simulink model "ADU_Integration_Y2016_simulation"  (R2016b)
settings: Solver=FixedStepDiscrete  StartTime=240  StopTime=300  FixedStep=0.01  RelTol=1e-3  EnableMultiTasking=on
PostLoadFcn:
  | , if any(exist('dsrtsu_mdlpostloadfcn', 'file') == [2, 3, 6]), try dsrtsu_mdlpostloadfcn('Execute', bdroot); catch fprintf('Error in PostLoadFcn (dsrtsu_mdlpostloadfcn) for model "%s":\n %s\n', bdroot, lasterr); end, end,
InitFcn:
  | load 'data/chi2_dat';
  | load 'data/innerLine_struct';
  | load 'data/middleLine_struct';
  | load 'data/outerLine_struct';
  | load 'data/innerLine';
  | load 'data/middleLine';
  | load 'data/outerLine';
  | load 'data/landmarks_patac_schimmel_ccw';
  | load 'data/patac_navi_array';
  | load 'data/sensor';
  | load 'data/map_struct';
  | addpath map_src
  | Integration_Parameter;
  | load 'TestData_001';
values from neighbouring files (symbols this model uses):
  TestData_001 =     [TestData_001.mat]
undefined symbols (not defined in the file or in its folder): a, chi2_dat, innerLine, landmarks_patac_schimmel_ccw, middleLine, outerLine, patac_navi_array, StartNum
libraries: simulink x36, rtican x1
(part 8 of 20)

== system ADU_Integration_Y2016_simulation/Fusion_Model/Fusion_Block/Side_Fusion/Side_Fusion/Tracker_Update.Tracker_Filter.Update.Update ==
  Pre_x : Inport
  Pre_vx : Inport  Port=2
  Pre_y : Inport  Port=3
  Pre_vy : Inport  Port=4
  pre_p11 : Inport  Port=5
  pre_p12 : Inport  Port=6
  pre_p13 : Inport  Port=7
  pre_p14 : Inport  Port=8
  pre_p21 : Inport  Port=9
  pre_p22 : Inport  Port=10
  pre_p23 : Inport  Port=11
  pre_p24 : Inport  Port=12
  pre_p31 : Inport  Port=13
  pre_p32 : Inport  Port=14
  pre_p33 : Inport  Port=15
  pre_p34 : Inport  Port=16
  pre_p41 : Inport  Port=17
  pre_p42 : Inport  Port=18
  pre_p43 : Inport  Port=19
  pre_p44 : Inport  Port=20
  mk : Inport  Port=21
  m00 : Inport  Port=22
  m01 : Inport  Port=23
  m2 : Inport  Port=24
  m10 : Inport  Port=25
  m11 : Inport  Port=26
  m12 : Inport  Port=27
  m20 : Inport  Port=28
  m21 : Inport  Port=29
  m22 : Inport  Port=30
  Pt0 : Inport  Port=31
  f : TriggerPort  TriggerType=function-call  VariantControl=Variant
      settings: CopyFcn=Stateflow.SLINSF.SimulinkMan.removeBlockPreDeleteFcn  PreDeleteFcn=Stateflow.SLINSF.SimulinkMan.unsafePredeleteFcn
  Model_Update : Subsystem
  RangeX : Outport
  VelX : Outport  Port=2
  RangeY : Outport  Port=3
  VelY : Outport  Port=4
  P11 : Outport  Port=5
  P12 : Outport  Port=6
  P13 : Outport  Port=7
  P14 : Outport  Port=8
  P21 : Outport  Port=9
  P22 : Outport  Port=10
  P23 : Outport  Port=11
  P24 : Outport  Port=12
  P31 : Outport  Port=13
  P32 : Outport  Port=14
  P33 : Outport  Port=15
  P34 : Outport  Port=16
  P41 : Outport  Port=17
  P42 : Outport  Port=18
  P43 : Outport  Port=19
  P44 : Outport  Port=20
  wires:
  Model_Update/1(RangeX) -> RangeX/1
  Model_Update/2(VelX) -> VelX/1
  Model_Update/3(RangeY) -> RangeY/1
  Model_Update/4(VelY) -> VelY/1
  Model_Update/5(P11) -> P11/1
  Model_Update/6(P12) -> P12/1
  Model_Update/7(P13) -> P13/1
  Model_Update/8(P14) -> P14/1
  Model_Update/9(P21) -> P21/1
  Model_Update/10(P22) -> P22/1
  Model_Update/11(P23) -> P23/1
  Model_Update/12(P24) -> P24/1
  Model_Update/13(P31) -> P31/1
  Model_Update/14(P32) -> P32/1
  Model_Update/15(P33) -> P33/1
  Model_Update/16(P34) -> P34/1
  Model_Update/17(P41) -> P41/1
  Model_Update/18(P42) -> P42/1
  Model_Update/19(P43) -> P43/1
  Model_Update/20(P44) -> P44/1
  pre_p41/1 -> Model_Update/17(pre_p41)
  pre_p33/1 -> Model_Update/15(pre_p33)
  pre_p34/1 -> Model_Update/16(pre_p34)
  pre_p42/1 -> Model_Update/18(pre_p42)
  pre_p24/1 -> Model_Update/12(pre_p24)
  pre_p31/1 -> Model_Update/13(pre_p31)
  pre_p32/1 -> Model_Update/14(pre_p32)
  mk/1 -> Model_Update/21(mk)  "Measurement_Num"
  pre_p22/1 -> Model_Update/10(pre_p22)
  pre_p43/1 -> Model_Update/19(pre_p43)
  pre_p44/1 -> Model_Update/20(pre_p44)
  pre_p23/1 -> Model_Update/11(pre_p23)
  pre_p21/1 -> Model_Update/9(pre_p21)
  pre_p11/1 -> Model_Update/5(pre_p11)
  Pre_y/1 -> Model_Update/3(Pre_y)  "Pre_y"
  Pre_x/1 -> Model_Update/1(Pre_x)  "Pre_x"
  Pre_vx/1 -> Model_Update/2(Pre_vx)  "Pre_vx"
  Pre_vy/1 -> Model_Update/4(Pre_vy)  "Pre_vy"
  pre_p12/1 -> Model_Update/6(pre_p12)
  pre_p13/1 -> Model_Update/7(pre_p13)
  pre_p14/1 -> Model_Update/8(pre_p14)
  m00/1 -> Model_Update/22(m00)  "Measurement_1_Possible"
  m12/1 -> Model_Update/27(m12)  "Measurement_2_Y_Error"
  m2/1 -> Model_Update/24(m2)  "Measurement_1_Y_Error"
  m11/1 -> Model_Update/26(m11)  "Measurement_2_X_Error"
  m10/1 -> Model_Update/25(m10)  "Measurement_2_Possible"
  m01/1 -> Model_Update/23(m01)  "Measurement_1_X_Error"
  m20/1 -> Model_Update/28(m20)  "Measurement_3_Possible"
  m22/1 -> Model_Update/30(m22)  "Measurement_3_Y_Error"
  m21/1 -> Model_Update/29(m21)  "Measurement_3_X_Error"
  Pt0/1 -> Model_Update/31(Pt0)

== system ADU_Integration_Y2016_simulation/Fusion_Model/Fusion_Block/Global_Fusion/Fusion_Center/FusTrackPredict.Forecast/No_Zero1 ==
  In : Inport
  Abs : Abs
  Compare To Constant : simulink/Logic and Bit Operations/Compare To Constant  relop=>=  const=0.001  OutDataTypeStr=uint8
  Constant : Constant  Value=0.001
  Switch : Switch  Threshold=0.5
  Out : Outport
  wires:
  Constant/1 -> Switch/3
  Switch/1 -> Out/1
  Compare To Constant/1 -> Switch/2
  In/1 -> Switch/1, Abs/1
  Abs/1 -> Compare To Constant/1

== system ADU_Integration_Y2016_simulation/Fusion_Model/Fusion_Block/Global_Fusion/Fusion_Center/FusTrackPredict.Forecast/No_Zero2 ==
  In : Inport
  Abs : Abs
  Compare To Constant : simulink/Logic and Bit Operations/Compare To Constant  relop=>=  const=0.001  OutDataTypeStr=uint8
  Constant : Constant  Value=0.001
  Switch : Switch  Threshold=0.5
  Out : Outport
  wires:
  Abs/1 -> Compare To Constant/1
  In/1 -> Abs/1, Switch/1
  Compare To Constant/1 -> Switch/2
  Switch/1 -> Out/1
  Constant/1 -> Switch/3

== system ADU_Integration_Y2016_simulation/Fusion_Model/Fusion_Block/Global_Fusion/Fusion_Center/FusTrackPredict.Forecast/No_Zero3 ==
  In : Inport
  Abs : Abs
  Compare To Constant : simulink/Logic and Bit Operations/Compare To Constant  relop=>=  const=0.001  OutDataTypeStr=uint8
  Constant : Constant  Value=0.001
  Switch : Switch  Threshold=0.5
  Out : Outport
  wires:
  Constant/1 -> Switch/3
  Switch/1 -> Out/1
  Compare To Constant/1 -> Switch/2
  In/1 -> Switch/1, Abs/1
  Abs/1 -> Compare To Constant/1

== system ADU_Integration_Y2016_simulation/Fusion_Model/Fusion_Block/Global_Fusion/Fusion_Center/FusTrackPredict.Forecast/No_Zero4 ==
  In : Inport
  Abs : Abs
  Compare To Constant : simulink/Logic and Bit Operations/Compare To Constant  relop=>=  const=0.001  OutDataTypeStr=uint8
  Constant : Constant  Value=0.001
  Switch : Switch  Threshold=0.5
  Out : Outport
  wires:
  Abs/1 -> Compare To Constant/1
  In/1 -> Abs/1, Switch/1
  Compare To Constant/1 -> Switch/2
  Switch/1 -> Out/1
  Constant/1 -> Switch/3

== system ADU_Integration_Y2016_simulation/Fusion_Model/Fusion_Block/Global_Fusion/Fusion_Center/FusTrackPredict.Forecast/P_Gen ==
  pre_p11 : Inport
  pre_p12 : Inport  Port=2
  pre_p13 : Inport  Port=3
  pre_p14 : Inport  Port=4
  pre_p21 : Inport  Port=5
  pre_p22 : Inport  Port=6
  pre_p23 : Inport  Port=7
  pre_p24 : Inport  Port=8
  pre_p31 : Inport  Port=9
  pre_p32 : Inport  Port=10
  pre_p33 : Inport  Port=11
  pre_p34 : Inport  Port=12
  pre_p41 : Inport  Port=13
  pre_p42 : Inport  Port=14
  pre_p43 : Inport  Port=15
  pre_p44 : Inport  Port=16
  Add : Sum  Inputs=++++
  Gain : Gain  Gain=[1;0;0;0]  Multiplication=Matrix(K*u)
  Gain1 : Gain  Gain=[0;1;0;0]  Multiplication=Matrix(K*u)
  Gain2 : Gain  Gain=[0;0;1;0]  Multiplication=Matrix(K*u)
  Gain3 : Gain  Gain=[0;0;0;1]  Multiplication=Matrix(K*u)
  Math Function{1..4} (4 alike) : Math  Operator=transpose  SaturateOnIntegerOverflow=on
  Mux{,1..3} (4 alike) : Mux
  P_Pre[4x4] : Outport
  wires:
  Mux/1 -> Math Function2/1
  Math Function2/1 -> Gain/1
  Mux1/1 -> Math Function1/1
  Math Function1/1 -> Gain1/1
  Mux2/1 -> Math Function4/1
  Math Function4/1 -> Gain2/1
  Mux3/1 -> Math Function3/1
  Math Function3/1 -> Gain3/1
  Gain/1 -> Add/1
  Gain1/1 -> Add/2
  Gain2/1 -> Add/3
  Gain3/1 -> Add/4
  pre_p11/1 -> Mux/1
  pre_p12/1 -> Mux/2
  pre_p13/1 -> Mux/3
  pre_p14/1 -> Mux/4
  pre_p21/1 -> Mux1/1
  pre_p22/1 -> Mux1/2
  pre_p23/1 -> Mux1/3
  pre_p24/1 -> Mux1/4
  pre_p31/1 -> Mux2/1
  pre_p32/1 -> Mux2/2
  pre_p33/1 -> Mux2/3
  pre_p34/1 -> Mux2/4
  pre_p41/1 -> Mux3/1
  pre_p42/1 -> Mux3/2
  pre_p43/1 -> Mux3/3
  pre_p44/1 -> Mux3/4
  Add/1 -> P_Pre[4x4]/1

== system ADU_Integration_Y2016_simulation/Fusion_Model/Fusion_Block/Global_Fusion/Fusion_Center/FusTrackPredict.Forecast/Predict ==
  DataIn : Inport
  Bus Creator1 : BusCreator  Inputs=2
  F : Subsystem
  State_PreTime : Subsystem
  DataOut : Outport
  wires:
  DataIn/1 -> F/1(DataIn), State_PreTime/1(Source)  "Z_Mea"
  State_PreTime/1(X_k) -> Bus Creator1/1  "X_k[4x1]"
  F/1(F) -> Bus Creator1/2  "F[4x4]"
  Bus Creator1/1 -> DataOut/1

== system ADU_Integration_Y2016_simulation/Fusion_Model/Fusion_Block/Global_Fusion/Fusion_Center/FusTrackPredict.Forecast/Predict_X_P ==
  In : Inport
  P_k : Inport  Port=2
  Bus Creator : BusCreator  Inputs=3
  Bus Selector : BusSelector  OutputSignals=F[4x4],X_k[4x1]
  Bus Selector1 : BusSelector  OutputSignals=F[4x4],F[4x4]
  Math Function : Math  Operator=transpose  SaturateOnIntegerOverflow=on
  Product : Product  Multiplication=Matrix(*)  RndMeth=Zero
  Product1 : Product  Inputs=3  Multiplication=Matrix(*)  RndMeth=Zero
  Q : Constant  Value=[0.01 0 0 0;0 0.01 0 0;0 0 0.01 0;0 0 0 0.01]
  Subtract2 : Sum
  DataOut : Outport
  wires:
  In/1 -> Bus Selector/1, Bus Selector1/1, Bus Creator/3  "Signal_temp"
  Bus Selector/1 -> Product/1  "<F[4x4]>"
  Bus Selector/2 -> Product/2  "<X_k[4x1]>"
  P_k/1 -> Product1/2
  Bus Selector1/1 -> Product1/1  "<F[4x4]>"
  Bus Selector1/2 -> Math Function/1  "<F[4x4]>"
  Math Function/1 -> Product1/3
  Product/1 -> Bus Creator/1  "x_predict[4x1]"
  Subtract2/1 -> Bus Creator/2  "P_predict"
  Bus Creator/1 -> DataOut/1
  Product1/1 -> Subtract2/1  "P_predict"
  Q/1 -> Subtract2/2

== system ADU_Integration_Y2016_simulation/Fusion_Model/Fusion_Block/Global_Fusion/Fusion_Center/FusTrackUpdate.MDCal/No_Zero1 ==
  In : Inport
  Abs : Abs
  Compare To Constant : simulink/Logic and Bit Operations/Compare To Constant  relop=>=  const=0.001  OutDataTypeStr=uint8
  Constant : Constant  Value=0.001
  Switch : Switch  Threshold=0.5
  Out : Outport
  wires:
  Constant/1 -> Switch/3
  Switch/1 -> Out/1
  Compare To Constant/1 -> Switch/2
  In/1 -> Switch/1, Abs/1
  Abs/1 -> Compare To Constant/1

== system ADU_Integration_Y2016_simulation/Fusion_Model/Fusion_Block/Global_Fusion/Fusion_Center/FusTrackUpdate.MDCal/No_Zero2 ==
  In : Inport
  Abs : Abs
  Compare To Constant : simulink/Logic and Bit Operations/Compare To Constant  relop=>=  const=0.001  OutDataTypeStr=uint8
  Constant : Constant  Value=0.001
  Switch : Switch  Threshold=0.5
  Out : Outport
  wires:
  Abs/1 -> Compare To Constant/1
  In/1 -> Abs/1, Switch/1
  Compare To Constant/1 -> Switch/2
  Switch/1 -> Out/1
  Constant/1 -> Switch/3

== system ADU_Integration_Y2016_simulation/Fusion_Model/Fusion_Block/Global_Fusion/Fusion_Center/FusTrackUpdate.MDCal/No_Zero3 ==
  In : Inport
  Abs : Abs
  Compare To Constant : simulink/Logic and Bit Operations/Compare To Constant  relop=>=  const=0.001  OutDataTypeStr=uint8
  Constant : Constant  Value=0.001
  Switch : Switch  Threshold=0.5
  Out : Outport
  wires:
  Constant/1 -> Switch/3
  Switch/1 -> Out/1
  Compare To Constant/1 -> Switch/2
  In/1 -> Switch/1, Abs/1
  Abs/1 -> Compare To Constant/1

== system ADU_Integration_Y2016_simulation/Fusion_Model/Fusion_Block/Global_Fusion/Fusion_Center/FusTrackUpdate.MDCal/No_Zero4 ==
  In : Inport
  Abs : Abs
  Compare To Constant : simulink/Logic and Bit Operations/Compare To Constant  relop=>=  const=0.001  OutDataTypeStr=uint8
  Constant : Constant  Value=0.001
  Switch : Switch  Threshold=0.5
  Out : Outport
  wires:
  Abs/1 -> Compare To Constant/1
  In/1 -> Abs/1, Switch/1
  Compare To Constant/1 -> Switch/2
  Switch/1 -> Out/1
  Constant/1 -> Switch/3

== system ADU_Integration_Y2016_simulation/Fusion_Model/Fusion_Block/Global_Fusion/Fusion_Center/FusTrackUpdate.MDCal/Subsystem ==
  R11 : Inport
  R12 : Inport  Port=2
  R21 : Inport  Port=3
  R22 : Inport  Port=4
  Add : Sum
  Gain : Gain  Gain=[1;0]  Multiplication=Matrix(K*u)
  Gain1 : Gain  Gain=[0;1]  Multiplication=Matrix(K*u)
  Math Function1 : Math  Operator=transpose  SaturateOnIntegerOverflow=on
  Math Function2 : Math  Operator=transpose  SaturateOnIntegerOverflow=on
  Mux2 : Mux  Inputs=2
  Mux3 : Mux  Inputs=2
  R[2x2] : Outport
  wires:
  R21/1 -> Mux3/1
  Gain1/1 -> Add/2
  Math Function1/1 -> Gain1/1
  R22/1 -> Mux3/2
  Mux3/1 -> Math Function1/1
  Mux2/1 -> Math Function2/1
  Gain/1 -> Add/1
  Math Function2/1 -> Gain/1
  Add/1 -> R[2x2]/1
  R11/1 -> Mux2/1
  R12/1 -> Mux2/2

== system ADU_Integration_Y2016_simulation/Fusion_Model/Fusion_Block/Global_Fusion/Fusion_Center/FusTrackUpdate.MDCal/W_Gen ==
  R11 : Inport
  R12 : Inport  Port=2
  R13 : Inport  Port=3
  R14 : Inport  Port=4
  R21 : Inport  Port=5
  R22 : Inport  Port=6
  R23 : Inport  Port=7
  R24 : Inport  Port=8
  R31 : Inport  Port=9
  R32 : Inport  Port=10
  R33 : Inport  Port=11
  R34 : Inport  Port=12
  R41 : Inport  Port=13
  R42 : Inport  Port=14
  R43 : Inport  Port=15
  R44 : Inport  Port=16
  Add : Sum  Inputs=++++
  Gain : Gain  Gain=[1;0;0;0]  Multiplication=Matrix(K*u)
  Gain1 : Gain  Gain=[0;1;0;0]  Multiplication=Matrix(K*u)
  Gain2 : Gain  Gain=[0;0;1;0]  Multiplication=Matrix(K*u)
  Gain3 : Gain  Gain=[0;0;0;1]  Multiplication=Matrix(K*u)
  Math Function{1..4} (4 alike) : Math  Operator=transpose  SaturateOnIntegerOverflow=on
  Mux{,1..3} (4 alike) : Mux
  P_Pre : Outport
  wires:
  Mux/1 -> Math Function2/1
  Math Function2/1 -> Gain/1
  Mux1/1 -> Math Function1/1
  Math Function1/1 -> Gain1/1
  Mux2/1 -> Math Function4/1
  Math Function4/1 -> Gain2/1
  Mux3/1 -> Math Function3/1
  Math Function3/1 -> Gain3/1
  Gain/1 -> Add/1
  Gain1/1 -> Add/2
  Gain2/1 -> Add/3
  Gain3/1 -> Add/4
  R11/1 -> Mux/1
  R12/1 -> Mux/2
  R13/1 -> Mux/3
  R14/1 -> Mux/4
  R21/1 -> Mux1/1
  R22/1 -> Mux1/2
  R23/1 -> Mux1/3
  R24/1 -> Mux1/4
  R31/1 -> Mux2/1
  R32/1 -> Mux2/2
  R33/1 -> Mux2/3
  R34/1 -> Mux2/4
  R41/1 -> Mux3/1
  R42/1 -> Mux3/2
  R43/1 -> Mux3/3
  R44/1 -> Mux3/4
  Add/1 -> P_Pre/1

== system ADU_Integration_Y2016_simulation/Fusion_Model/Fusion_Block/Global_Fusion/Fusion_Center/FusTrackUpdate.Update/No_Zero1 ==
  In : Inport
  Abs : Abs
  Compare To Constant : simulink/Logic and Bit Operations/Compare To Constant  relop=>=  const=0.001  OutDataTypeStr=uint8
  Constant : Constant  Value=0.001
  Switch : Switch  Threshold=0.5
  Out : Outport
  wires:
  Abs/1 -> Compare To Constant/1
  In/1 -> Abs/1, Switch/1
  Compare To Constant/1 -> Switch/2
  Switch/1 -> Out/1
  Constant/1 -> Switch/3

== system ADU_Integration_Y2016_simulation/Fusion_Model/Fusion_Block/Global_Fusion/Fusion_Center/FusTrackUpdate.Update/No_Zero2 ==
  In : Inport
  Abs : Abs
  Compare To Constant : simulink/Logic and Bit Operations/Compare To Constant  relop=>=  const=0.001  OutDataTypeStr=uint8
  Constant : Constant  Value=0.001
  Switch : Switch  Threshold=0.5
  Out : Outport
  wires:
  Constant/1 -> Switch/3
  Switch/1 -> Out/1
  Compare To Constant/1 -> Switch/2
  In/1 -> Switch/1, Abs/1
  Abs/1 -> Compare To Constant/1

== system ADU_Integration_Y2016_simulation/Fusion_Model/Fusion_Block/Global_Fusion/Fusion_Center/FusTrackUpdate.Update/No_Zero3 ==
  In : Inport
  Abs : Abs
  Compare To Constant : simulink/Logic and Bit Operations/Compare To Constant  relop=>=  const=0.001  OutDataTypeStr=uint8
  Constant : Constant  Value=0.001
  Switch : Switch  Threshold=0.5
  Out : Outport
  wires:
  Abs/1 -> Compare To Constant/1
  In/1 -> Abs/1, Switch/1
  Compare To Constant/1 -> Switch/2
  Switch/1 -> Out/1
  Constant/1 -> Switch/3

== system ADU_Integration_Y2016_simulation/Fusion_Model/Fusion_Block/Global_Fusion/Fusion_Center/FusTrackUpdate.Update/No_Zero4 ==
  In : Inport
  Abs : Abs
  Compare To Constant : simulink/Logic and Bit Operations/Compare To Constant  relop=>=  const=0.001  OutDataTypeStr=uint8
  Constant : Constant  Value=0.001
  Switch : Switch  Threshold=0.5
  Out : Outport
  wires:
  Constant/1 -> Switch/3
  Switch/1 -> Out/1
  Compare To Constant/1 -> Switch/2
  In/1 -> Switch/1, Abs/1
  Abs/1 -> Compare To Constant/1

== system ADU_Integration_Y2016_simulation/Fusion_Model/Fusion_Block/Global_Fusion/Fusion_Center/FusTrackUpdate.Update/P_Gen ==
  pre_p11 : Inport
  pre_p12 : Inport  Port=2
  pre_p13 : Inport  Port=3
  pre_p14 : Inport  Port=4
  pre_p21 : Inport  Port=5
  pre_p22 : Inport  Port=6
  pre_p23 : Inport  Port=7
  pre_p24 : Inport  Port=8
  pre_p31 : Inport  Port=9
  pre_p32 : Inport  Port=10
  pre_p33 : Inport  Port=11
  pre_p34 : Inport  Port=12
  pre_p41 : Inport  Port=13
  pre_p42 : Inport  Port=14
  pre_p43 : Inport  Port=15
  pre_p44 : Inport  Port=16
  Add : Sum  Inputs=++++
  Gain : Gain  Gain=[1;0;0;0]  Multiplication=Matrix(K*u)
  Gain1 : Gain  Gain=[0;1;0;0]  Multiplication=Matrix(K*u)
  Gain2 : Gain  Gain=[0;0;1;0]  Multiplication=Matrix(K*u)
  Gain3 : Gain  Gain=[0;0;0;1]  Multiplication=Matrix(K*u)
  Math Function{1..4} (4 alike) : Math  Operator=transpose  SaturateOnIntegerOverflow=on
  Mux{,1..3} (4 alike) : Mux
  P_Pre : Outport
  wires:
  Mux/1 -> Math Function2/1
  Math Function2/1 -> Gain/1
  Mux1/1 -> Math Function1/1
  Math Function1/1 -> Gain1/1
  Mux2/1 -> Math Function4/1
  Math Function4/1 -> Gain2/1
  Mux3/1 -> Math Function3/1
  Math Function3/1 -> Gain3/1
  Gain/1 -> Add/1
  Gain1/1 -> Add/2
  Gain2/1 -> Add/3
  Gain3/1 -> Add/4
  pre_p11/1 -> Mux/1
  pre_p12/1 -> Mux/2
  pre_p13/1 -> Mux/3
  pre_p14/1 -> Mux/4
  pre_p21/1 -> Mux1/1
  pre_p22/1 -> Mux1/2
  pre_p23/1 -> Mux1/3
  pre_p24/1 -> Mux1/4
  pre_p31/1 -> Mux2/1
  pre_p32/1 -> Mux2/2
  pre_p33/1 -> Mux2/3
  pre_p34/1 -> Mux2/4
  pre_p41/1 -> Mux3/1
  pre_p42/1 -> Mux3/2
  pre_p43/1 -> Mux3/3
  pre_p44/1 -> Mux3/4
  Add/1 -> P_Pre/1

== system ADU_Integration_Y2016_simulation/Fusion_Model/Fusion_Block/Global_Fusion/Fusion_Center/FusTrackUpdate.Update/Predict ==
  DataIn : Inport
  Bus Creator1 : BusCreator  Inputs=3
  H : Constant  Value=[1 0 0 0;0 0 1 0]
  Measurement : Subsystem
  State_PreTime : Subsystem
  DataOut : Outport
  wires:
  DataIn/1 -> Measurement/1(Source), State_PreTime/1(Source)
  State_PreTime/1(X_k) -> Bus Creator1/1  "X_k"
  Measurement/1(Z_k) -> Bus Creator1/2  "Z_Mea"
  H/1 -> Bus Creator1/3  "H"
  Bus Creator1/1 -> DataOut/1

== system ADU_Integration_Y2016_simulation/Fusion_Model/Fusion_Block/Global_Fusion/Fusion_Center/FusTrackUpdate.Update/Predict_X_P ==
  In : Inport
  P_k : Inport  Port=2
  Bus Creator : BusCreator  Inputs=3
  Bus Selector : BusSelector  OutputSignals=X_k
  Gain : Gain
  DataOut : Outport
  wires:
  In/1 -> Bus Selector/1, Bus Creator/3  "Signal_temp"
  Bus Creator/1 -> DataOut/1
  Bus Selector/1 -> Gain/1  "<X_k>"
  P_k/1 -> Bus Creator/2  "P_predict"
  Gain/1 -> Bus Creator/1  "x_predict"

== system ADU_Integration_Y2016_simulation/Fusion_Model/Fusion_Block/Global_Fusion/Fusion_Center/FusTrackUpdate.Update/R_Cov_Gen ==
  R11 : Inport
  R12 : Inport  Port=2
  R21 : Inport  Port=3
  R22 : Inport  Port=4
  Add : Sum
  Gain : Gain  Gain=[1;0]  Multiplication=Matrix(K*u)
  Gain1 : Gain  Gain=[0;1]  Multiplication=Matrix(K*u)
  Math Function1 : Math  Operator=transpose  SaturateOnIntegerOverflow=on
  Math Function2 : Math  Operator=transpose  SaturateOnIntegerOverflow=on
  Mux : Mux  Inputs=2
  Mux1 : Mux  Inputs=2
  Cov_R_Measuerment : Outport
  wires:
  Add/1 -> Cov_R_Measuerment/1
  R22/1 -> Mux1/2
  R21/1 -> Mux1/1
  R12/1 -> Mux/2
  R11/1 -> Mux/1
  Gain1/1 -> Add/2
  Gain/1 -> Add/1
  Math Function1/1 -> Gain1/1
  Mux1/1 -> Math Function1/1
  Math Function2/1 -> Gain/1
  Mux/1 -> Math Function2/1

== system ADU_Integration_Y2016_simulation/Fusion_Model/Fusion_Block/Global_Fusion/Fusion_Center/FusTrackUpdate.Update/X_new ==
  note: 2X1
  note: 4X1
  note: 2X4
  note: 4X4
  note: 2X4
  note: 4X4
  note: 2X4
  W_k : Inport
  Data_In : Inport  Port=2
  Bus Selector : BusSelector  OutputSignals=P_predict,Signal_temp.H,Signal_temp.H,P_predict,Signal_temp.H
  Bus Selector1 : BusSelector  OutputSignals=Signal_temp.Z_Mea,Signal_temp.H,x_predict,x_predict
  Divide : Product  Inputs=*/  Multiplication=Matrix(*)
  Divide1 : Product  Inputs=**  Multiplication=Matrix(*)
  Divide2 : Product  Inputs=***  Multiplication=Matrix(*)
  Divide3 : Product  Inputs=**  Multiplication=Matrix(*)
  Divide4 : Product  Inputs=**  Multiplication=Matrix(*)
  Math Function : Math  Operator=transpose  SaturateOnIntegerOverflow=on
  Math Function1 : Math  Operator=transpose  SaturateOnIntegerOverflow=on
  Subtract : Sum
  Subtract1 : Sum
  Subtract2 : Sum  Inputs=+-
  X_update : Outport
  K : Outport  Port=2
  wires:
  Data_In/1 -> Bus Selector1/1, Bus Selector/1
  Bus Selector/1 -> Divide1/1  "<P_predict>"
  Bus Selector/2 -> Math Function1/1  "<H>"
  Bus Selector/5 -> Math Function/1  "<H>"
  Math Function/1 -> Divide2/3  "4X2"
  Bus Selector/4 -> Divide2/2  "<P_predict>"
  Bus Selector/3 -> Divide2/1  "<H>"
  Divide1/1 -> Divide/1  "4X2"
  Divide2/1 -> Subtract/1
  W_k/1 -> Subtract/2  "2X2"
  Subtract/1 -> Divide/2  "2X2"
  Bus Selector1/1 -> Subtract2/1  "<Z_Mea>"
  Bus Selector1/2 -> Divide3/1  "<H>"
  Divide3/1 -> Subtract2/2
  Bus Selector1/3 -> Divide3/2  "<x_predict>"
  Subtract2/1 -> Divide4/2
  Divide/1 -> Divide4/1, K/1  "K[4X2]"
  Divide4/1 -> Subtract1/1  "4X1"
  Bus Selector1/4 -> Subtract1/2  "<x_predict>"
  Subtract1/1 -> X_update/1
  Math Function1/1 -> Divide1/2  "4X2"

== system ADU_Integration_Y2016_simulation/Fusion_Model/Fusion_Block/Side_Fusion/Side_Fusion/FusTrackPredict.Forecast/No_Zero1 ==
  In : Inport
  Abs : Abs
  Compare To Constant : simulink/Logic and Bit Operations/Compare To Constant  relop=>=  const=0.001  OutDataTypeStr=uint8
  Constant : Constant  Value=0.001
  Switch : Switch  Threshold=0.5
  Out : Outport
  wires:
  Constant/1 -> Switch/3
  Switch/1 -> Out/1
  Compare To Constant/1 -> Switch/2
  In/1 -> Switch/1, Abs/1
  Abs/1 -> Compare To Constant/1

== system ADU_Integration_Y2016_simulation/Fusion_Model/Fusion_Block/Side_Fusion/Side_Fusion/FusTrackPredict.Forecast/No_Zero2 ==
  In : Inport
  Abs : Abs
  Compare To Constant : simulink/Logic and Bit Operations/Compare To Constant  relop=>=  const=0.001  OutDataTypeStr=uint8
  Constant : Constant  Value=0.001
  Switch : Switch  Threshold=0.5
  Out : Outport
  wires:
  Abs/1 -> Compare To Constant/1
  In/1 -> Abs/1, Switch/1
  Compare To Constant/1 -> Switch/2
  Switch/1 -> Out/1
  Constant/1 -> Switch/3

== system ADU_Integration_Y2016_simulation/Fusion_Model/Fusion_Block/Side_Fusion/Side_Fusion/FusTrackPredict.Forecast/No_Zero3 ==
  In : Inport
  Abs : Abs
  Compare To Constant : simulink/Logic and Bit Operations/Compare To Constant  relop=>=  const=0.001  OutDataTypeStr=uint8
  Constant : Constant  Value=0.001
  Switch : Switch  Threshold=0.5
  Out : Outport
  wires:
  Constant/1 -> Switch/3
  Switch/1 -> Out/1
  Compare To Constant/1 -> Switch/2
  In/1 -> Switch/1, Abs/1
  Abs/1 -> Compare To Constant/1

== system ADU_Integration_Y2016_simulation/Fusion_Model/Fusion_Block/Side_Fusion/Side_Fusion/FusTrackPredict.Forecast/No_Zero4 ==
  In : Inport
  Abs : Abs
  Compare To Constant : simulink/Logic and Bit Operations/Compare To Constant  relop=>=  const=0.001  OutDataTypeStr=uint8
  Constant : Constant  Value=0.001
  Switch : Switch  Threshold=0.5
  Out : Outport
  wires:
  Abs/1 -> Compare To Constant/1
  In/1 -> Abs/1, Switch/1
  Compare To Constant/1 -> Switch/2
  Switch/1 -> Out/1
  Constant/1 -> Switch/3

== system ADU_Integration_Y2016_simulation/Fusion_Model/Fusion_Block/Side_Fusion/Side_Fusion/FusTrackPredict.Forecast/P_Gen ==
  pre_p11 : Inport
  pre_p12 : Inport  Port=2
  pre_p13 : Inport  Port=3
  pre_p14 : Inport  Port=4
  pre_p21 : Inport  Port=5
  pre_p22 : Inport  Port=6
  pre_p23 : Inport  Port=7
  pre_p24 : Inport  Port=8
  pre_p31 : Inport  Port=9
  pre_p32 : Inport  Port=10
  pre_p33 : Inport  Port=11
  pre_p34 : Inport  Port=12
  pre_p41 : Inport  Port=13
  pre_p42 : Inport  Port=14
  pre_p43 : Inport  Port=15
  pre_p44 : Inport  Port=16
  Add : Sum  Inputs=++++
  Gain : Gain  Gain=[1;0;0;0]  Multiplication=Matrix(K*u)
  Gain1 : Gain  Gain=[0;1;0;0]  Multiplication=Matrix(K*u)
  Gain2 : Gain  Gain=[0;0;1;0]  Multiplication=Matrix(K*u)
  Gain3 : Gain  Gain=[0;0;0;1]  Multiplication=Matrix(K*u)
  Math Function{1..4} (4 alike) : Math  Operator=transpose  SaturateOnIntegerOverflow=on
  Mux{,1..3} (4 alike) : Mux
  P_Pre[4x4] : Outport
  wires:
  Mux/1 -> Math Function2/1
  Math Function2/1 -> Gain/1
  Mux1/1 -> Math Function1/1
  Math Function1/1 -> Gain1/1
  Mux2/1 -> Math Function4/1
  Math Function4/1 -> Gain2/1
  Mux3/1 -> Math Function3/1
  Math Function3/1 -> Gain3/1
  Gain/1 -> Add/1
  Gain1/1 -> Add/2
  Gain2/1 -> Add/3
  Gain3/1 -> Add/4
  pre_p11/1 -> Mux/1
  pre_p12/1 -> Mux/2
  pre_p13/1 -> Mux/3
  pre_p14/1 -> Mux/4
  pre_p21/1 -> Mux1/1
  pre_p22/1 -> Mux1/2
  pre_p23/1 -> Mux1/3
  pre_p24/1 -> Mux1/4
  pre_p31/1 -> Mux2/1
  pre_p32/1 -> Mux2/2
  pre_p33/1 -> Mux2/3
  pre_p34/1 -> Mux2/4
  pre_p41/1 -> Mux3/1
  pre_p42/1 -> Mux3/2
  pre_p43/1 -> Mux3/3
  pre_p44/1 -> Mux3/4
  Add/1 -> P_Pre[4x4]/1

== system ADU_Integration_Y2016_simulation/Fusion_Model/Fusion_Block/Side_Fusion/Side_Fusion/FusTrackPredict.Forecast/Predict ==
  DataIn : Inport
  Bus Creator1 : BusCreator  Inputs=2
  F : Subsystem
  State_PreTime : Subsystem
  DataOut : Outport
  wires:
  DataIn/1 -> F/1(DataIn), State_PreTime/1(Source)  "Z_Mea"
  State_PreTime/1(X_k) -> Bus Creator1/1  "X_k[4x1]"
  F/1(F) -> Bus Creator1/2  "F[4x4]"
  Bus Creator1/1 -> DataOut/1

== system ADU_Integration_Y2016_simulation/Fusion_Model/Fusion_Block/Side_Fusion/Side_Fusion/FusTrackPredict.Forecast/Predict_X_P ==
  In : Inport
  P_k : Inport  Port=2
  Bus Creator : BusCreator  Inputs=3
  Bus Selector : BusSelector  OutputSignals=F[4x4],X_k[4x1]
  Bus Selector1 : BusSelector  OutputSignals=F[4x4],F[4x4]
  Math Function : Math  Operator=transpose  SaturateOnIntegerOverflow=on
  Product : Product  Multiplication=Matrix(*)  RndMeth=Zero
  Product1 : Product  Inputs=3  Multiplication=Matrix(*)  RndMeth=Zero
  Q : Constant  Value=[0.01 0 0 0;0 0.01 0 0;0 0 0.01 0;0 0 0 0.01]
  Subtract2 : Sum
  DataOut : Outport
  wires:
  In/1 -> Bus Selector/1, Bus Selector1/1, Bus Creator/3  "Signal_temp"
  Bus Selector/1 -> Product/1  "<F[4x4]>"
  Bus Selector/2 -> Product/2  "<X_k[4x1]>"
  P_k/1 -> Product1/2
  Bus Selector1/1 -> Product1/1  "<F[4x4]>"
  Bus Selector1/2 -> Math Function/1  "<F[4x4]>"
  Math Function/1 -> Product1/3
  Product/1 -> Bus Creator/1  "x_predict[4x1]"
  Subtract2/1 -> Bus Creator/2  "P_predict"
  Bus Creator/1 -> DataOut/1
  Product1/1 -> Subtract2/1  "P_predict"
  Q/1 -> Subtract2/2

== system ADU_Integration_Y2016_simulation/Fusion_Model/Fusion_Block/Side_Fusion/Side_Fusion/G_cal/Cal_1 ==
  Stj : Inport
  Bus Selector : BusSelector  OutputSignals=11,22,21,12
  Constant : Constant
  Divide1 : Product  Inputs=**
  Divide2 : Product  Inputs=**
  Divide3 : Product  Inputs=**
  Sqrt1 : Math  Operator=sqrt  OutputSignalType=real  SaturateOnIntegerOverflow=on
  Subsystem1 : Subsystem
  Subtract3 : Sum  Inputs=+-
  sqrt_det_Stj : Outport
  wires:
  Stj/1 -> Subsystem1/1(Stj)
  Subsystem1/1(Stj_signal) -> Bus Selector/1
  Divide2/1 -> Subtract3/2
  Bus Selector/1 -> Divide1/1  "<11>"
  Bus Selector/4 -> Divide2/2  "<12>"
  Bus Selector/3 -> Divide2/1  "<21>"
  Divide1/1 -> Subtract3/1
  Bus Selector/2 -> Divide1/2  "<22>"
  Sqrt1/1 -> sqrt_det_Stj/1
  Subtract3/1 -> Divide3/1
  Constant/1 -> Divide3/2
  Divide3/1 -> Sqrt1/1

== system ADU_Integration_Y2016_simulation/Fusion_Model/Fusion_Block/Side_Fusion/Side_Fusion/G_cal/No_Zero1 ==
  In : Inport
  Abs : Abs
  Compare To Constant : simulink/Logic and Bit Operations/Compare To Constant  relop=>=  const=0.001  OutDataTypeStr=uint8
  Constant : Constant  Value=0.001
  Switch : Switch  Threshold=0.5
  Out : Outport
  wires:
  Constant/1 -> Switch/3
  Switch/1 -> Out/1
  Compare To Constant/1 -> Switch/2
  In/1 -> Switch/1, Abs/1
  Abs/1 -> Compare To Constant/1

== system ADU_Integration_Y2016_simulation/Fusion_Model/Fusion_Block/Side_Fusion/Side_Fusion/G_cal/No_Zero2 ==
  In : Inport
  Abs : Abs
  Compare To Constant : simulink/Logic and Bit Operations/Compare To Constant  relop=>=  const=0.001  OutDataTypeStr=uint8
  Constant : Constant  Value=0.001
  Switch : Switch  Threshold=0.5
  Out : Outport
  wires:
  Abs/1 -> Compare To Constant/1
  In/1 -> Abs/1, Switch/1
  Compare To Constant/1 -> Switch/2
  Switch/1 -> Out/1
  Constant/1 -> Switch/3

== system ADU_Integration_Y2016_simulation/Fusion_Model/Fusion_Block/Side_Fusion/Side_Fusion/G_cal/No_Zero3 ==
  In : Inport
  Abs : Abs
  Compare To Constant : simulink/Logic and Bit Operations/Compare To Constant  relop=>=  const=0.001  OutDataTypeStr=uint8
  Constant : Constant  Value=0.001
  Switch : Switch  Threshold=0.5
  Out : Outport
  wires:
  Constant/1 -> Switch/3
  Switch/1 -> Out/1
  Compare To Constant/1 -> Switch/2
  In/1 -> Switch/1, Abs/1
  Abs/1 -> Compare To Constant/1

== system ADU_Integration_Y2016_simulation/Fusion_Model/Fusion_Block/Side_Fusion/Side_Fusion/G_cal/No_Zero4 ==
  In : Inport
  Abs : Abs
  Compare To Constant : simulink/Logic and Bit Operations/Compare To Constant  relop=>=  const=0.001  OutDataTypeStr=uint8
  Constant : Constant  Value=0.001
  Switch : Switch  Threshold=0.5
  Out : Outport
  wires:
  Abs/1 -> Compare To Constant/1
  In/1 -> Abs/1, Switch/1
  Compare To Constant/1 -> Switch/2
  Switch/1 -> Out/1
  Constant/1 -> Switch/3

== system ADU_Integration_Y2016_simulation/Fusion_Model/Fusion_Block/Side_Fusion/Side_Fusion/G_cal/No_Zero5 ==
  In : Inport
  Abs : Abs
  Compare To Constant : simulink/Logic and Bit Operations/Compare To Constant  relop=>=  const=0.001  OutDataTypeStr=uint8
  Constant : Constant  Value=0.001
  Switch : Switch  Threshold=0.5
  Out : Outport
  wires:
  Constant/1 -> Switch/3
  Switch/1 -> Out/1
  Compare To Constant/1 -> Switch/2
  In/1 -> Switch/1, Abs/1
  Abs/1 -> Compare To Constant/1

== system ADU_Integration_Y2016_simulation/Fusion_Model/Fusion_Block/Side_Fusion/Side_Fusion/G_cal/No_Zero6 ==
  In : Inport
  Abs : Abs
  Compare To Constant : simulink/Logic and Bit Operations/Compare To Constant  relop=>=  const=0.001  OutDataTypeStr=uint8
  Constant : Constant  Value=0.001
  Switch : Switch  Threshold=0.5
  Out : Outport
  wires:
  Abs/1 -> Compare To Constant/1
  In/1 -> Abs/1, Switch/1
  Compare To Constant/1 -> Switch/2
  Switch/1 -> Out/1
  Constant/1 -> Switch/3

== system ADU_Integration_Y2016_simulation/Fusion_Model/Fusion_Block/Side_Fusion/Side_Fusion/G_cal/P_Gen ==
  p11 : Inport
  p12 : Inport  Port=2
  p13 : Inport  Port=3
  p14 : Inport  Port=4
  p21 : Inport  Port=5
  p22 : Inport  Port=6
  p23 : Inport  Port=7
  p24 : Inport  Port=8
  p31 : Inport  Port=9
  p32 : Inport  Port=10
  p33 : Inport  Port=11
  p34 : Inport  Port=12
  p41 : Inport  Port=13
  p42 : Inport  Port=14
  p43 : Inport  Port=15
  p44 : Inport  Port=16
  Add : Sum  Inputs=++++
  Gain : Gain  Gain=[1;0;0;0]  Multiplication=Matrix(K*u)
  Gain1 : Gain  Gain=[0;1;0;0]  Multiplication=Matrix(K*u)
  Gain2 : Gain  Gain=[0;0;1;0]  Multiplication=Matrix(K*u)
  Gain3 : Gain  Gain=[0;0;0;1]  Multiplication=Matrix(K*u)
  Math Function{1..4} (4 alike) : Math  Operator=transpose  SaturateOnIntegerOverflow=on
  Mux{,1..3} (4 alike) : Mux
  P[4x4] : Outport
  wires:
  Mux/1 -> Math Function2/1
  Math Function2/1 -> Gain/1
  Mux1/1 -> Math Function1/1
  Math Function1/1 -> Gain1/1
  Mux2/1 -> Math Function4/1
  Math Function4/1 -> Gain2/1
  Mux3/1 -> Math Function3/1
  Math Function3/1 -> Gain3/1
  Gain/1 -> Add/1
  Gain1/1 -> Add/2
  Gain2/1 -> Add/3
  Gain3/1 -> Add/4
  p11/1 -> Mux/1
  p12/1 -> Mux/2
  p13/1 -> Mux/3
  p14/1 -> Mux/4
  p21/1 -> Mux1/1
  p22/1 -> Mux1/2
  p23/1 -> Mux1/3
  p24/1 -> Mux1/4
  p31/1 -> Mux2/1
  p32/1 -> Mux2/2
  p33/1 -> Mux2/3
  p34/1 -> Mux2/4
  p41/1 -> Mux3/1
  p42/1 -> Mux3/2
  p43/1 -> Mux3/3
  p44/1 -> Mux3/4
  Add/1 -> P[4x4]/1

== system ADU_Integration_Y2016_simulation/Fusion_Model/Fusion_Block/Side_Fusion/Side_Fusion/G_cal/Subsystem ==
  R11 : Inport
  R12 : Inport  Port=2
  R21 : Inport  Port=3
  R22 : Inport  Port=4
  Add : Sum
  Gain1 : Gain  Gain=[0;1]  Multiplication=Matrix(K*u)
  Gain3 : Gain  Gain=[1;0]  Multiplication=Matrix(K*u)
  Math Function1 : Math  Operator=transpose  SaturateOnIntegerOverflow=on
  Math Function3 : Math  Operator=transpose  SaturateOnIntegerOverflow=on
  Mux1 : Mux  Inputs=2
  Mux3 : Mux  Inputs=2
  R[2X2] : Outport
  wires:
  Gain3/1 -> Add/1
  Gain1/1 -> Add/2
  Add/1 -> R[2X2]/1
  Mux1/1 -> Math Function1/1
  R21/1 -> Mux1/1
  R22/1 -> Mux1/2
  R12/1 -> Mux3/2
  R11/1 -> Mux3/1
  Math Function3/1 -> Gain3/1
  Mux3/1 -> Math Function3/1
  Math Function1/1 -> Gain1/1

== system ADU_Integration_Y2016_simulation/Fusion_Model/Fusion_Block/Side_Fusion/Side_Fusion/Tracker_Initial.VelocityMethod/Dmt ==
  x_t : Inport
  y_t : Inport  Port=2
  x_m : Inport  Port=3
  y_m : Inport  Port=4
  vx_max : Inport  Port=5
  vx_min : Inport  Port=6
  vy_max : Inport  Port=7
  vy_min : Inport  Port=8
  ts : Inport  Port=9
  Mux : Mux  Inputs=2
  X_vector_Gen : Subsystem
  Y_vector_Gen1 : Subsystem
  dmt[2x1] : Outport
  wires:
  y_m/1 -> Y_vector_Gen1/2(y_m)
  x_m/1 -> X_vector_Gen/2(x_m)
  vx_min/1 -> X_vector_Gen/4(vx_min)
  ts/1 -> Y_vector_Gen1/5(ts), X_vector_Gen/5(ts)
  vx_max/1 -> X_vector_Gen/3(vx_max)
  x_t/1 -> X_vector_Gen/1(x_t)
  vy_min/1 -> Y_vector_Gen1/4(vy_min)
  y_t/1 -> Y_vector_Gen1/1(y_t)
  vy_max/1 -> Y_vector_Gen1/3(vy_max)
  Mux/1 -> dmt[2x1]/1
  Y_vector_Gen1/1(y_vector) -> Mux/2
  X_vector_Gen/1(x_vector) -> Mux/1

== system ADU_Integration_Y2016_simulation/Fusion_Model/Fusion_Block/Side_Fusion/Side_Fusion/Tracker_Initial.VelocityMethod/R ==
  R11 : Inport
  R12 : Inport  Port=2
  R21 : Inport  Port=3
  R22 : Inport  Port=4
  Add : Sum
  Gain : Gain  Gain=[1;0]  Multiplication=Matrix(K*u)
  Gain1 : Gain  Gain=[0;1]  Multiplication=Matrix(K*u)
  Gain{2..5} (4 alike) : Gain  Gain=2
  Math Function1 : Math  Operator=transpose  SaturateOnIntegerOverflow=on
  Math Function2 : Math  Operator=transpose  SaturateOnIntegerOverflow=on
  Mux2 : Mux  Inputs=2
  Mux3 : Mux  Inputs=2
  R[2x2] : Outport
  wires:
  R21/1 -> Gain4/1
  Gain1/1 -> Add/2
  Math Function1/1 -> Gain1/1
  R22/1 -> Gain5/1
  Mux3/1 -> Math Function1/1
  Mux2/1 -> Math Function2/1
  Gain/1 -> Add/1
  Math Function2/1 -> Gain/1
  Add/1 -> R[2x2]/1
  R11/1 -> Gain2/1
  R12/1 -> Gain3/1
  Gain2/1 -> Mux2/1
  Gain3/1 -> Mux2/2
  Gain4/1 -> Mux3/1
  Gain5/1 -> Mux3/2

== system ADU_Integration_Y2016_simulation/Fusion_Model/Fusion_Block/Side_Fusion/Side_Fusion/Tracker_Initial.cos_cal/Reltive_Deg_Cal ==
  In1 : Inport
  Bus Selector1 : BusSelector  OutputSignals=a,b
  Bus Selector2 : BusSelector  OutputSignals=a,b,c,a,b
  Compare To Constant : simulink/Logic and Bit Operations/Compare To Constant  relop=~=  const=0  OutDataTypeStr=uint8
  Compare To Constant1 : simulink/Logic and Bit Operations/Compare To Constant  relop=>  const=0.01  OutDataTypeStr=uint8
  Compare To Constant2 : simulink/Logic and Bit Operations/Compare To Constant  relop=>  const=0.01  OutDataTypeStr=uint8
  Constant4 : Constant  Value=180
  Constant5 : Constant  Value=2
  Divide1 : Product  Inputs=**
  Divide2 : Product  Inputs=***
  Divide3 : Product  Inputs=*/
  Gain : Gain  Gain=180/pi
  Math Function2 : Math  Operator=square  SaturateOnIntegerOverflow=on
  Math Function3 : Math  Operator=square  SaturateOnIntegerOverflow=on
  Math Function4 : Math  Operator=square  SaturateOnIntegerOverflow=on
  Multiport Switch : MultiPortSwitch  DataPortOrder=Zero-based contiguous  Inputs=2  zeroidx=on
  Saturation2 : Saturate  UpperLimit=180  LowerLimit=0
  Side_Length_Cal : Subsystem
  Subtract2 : Sum  Inputs=++-
  Trigonometric Function1 : Trigonometry  Operator=acos
  Rel_Deg : Outport
  wires:
  Trigonometric Function1/1 -> Gain/1
  Subtract2/1 -> Divide3/1
  Bus Selector2/1 -> Math Function2/1  "<a>"
  Bus Selector2/2 -> Math Function3/1  "<b>"
  Divide3/1 -> Trigonometric Function1/1
  Divide2/1 -> Divide3/2
  Bus Selector2/5 -> Divide2/2  "<b>"
  Constant5/1 -> Divide2/3
  Side_Length_Cal/1(Out1) -> Bus Selector1/1, Bus Selector2/1
  In1/1 -> Side_Length_Cal/1(In1)
  Bus Selector2/3 -> Math Function4/1  "<c>"
  Bus Selector2/4 -> Divide2/1  "<a>"
  Math Function3/1 -> Subtract2/2
  Math Function2/1 -> Subtract2/1
  Math Function4/1 -> Subtract2/3
  Gain/1 -> Saturation2/1
  Saturation2/1 -> Multiport Switch/3
  Bus Selector1/2 -> Compare To Constant2/1  "<b>"
  Bus Selector1/1 -> Compare To Constant1/1  "<a>"
  Constant4/1 -> Multiport Switch/2
  Compare To Constant/1 -> Multiport Switch/1
  Multiport Switch/1 -> Rel_Deg/1
  Divide1/1 -> Compare To Constant/1
  Compare To Constant1/1 -> Divide1/1
  Compare To Constant2/1 -> Divide1/2

== system ADU_Integration_Y2016_simulation/Fusion_Model/Fusion_Block/Side_Fusion/Side_Fusion/Tracker_Update.Tracker_Filter.Update.Update/Model_Update ==
  Pre_x : Inport
  Pre_vx : Inport  Port=2
  Pre_y : Inport  Port=3
  Pre_vy : Inport  Port=4
  pre_p11 : Inport  Port=5
  pre_p12 : Inport  Port=6
  pre_p13 : Inport  Port=7
  pre_p14 : Inport  Port=8
  pre_p21 : Inport  Port=9
  pre_p22 : Inport  Port=10
  pre_p23 : Inport  Port=11
  pre_p24 : Inport  Port=12
  pre_p31 : Inport  Port=13
  pre_p32 : Inport  Port=14
  pre_p33 : Inport  Port=15
  pre_p34 : Inport  Port=16
  pre_p41 : Inport  Port=17
  pre_p42 : Inport  Port=18
  pre_p43 : Inport  Port=19
  pre_p44 : Inport  Port=20
  mk : Inport  Port=21
  m00 : Inport  Port=22
  m01 : Inport  Port=23
  m2 : Inport  Port=24
  m10 : Inport  Port=25
  m11 : Inport  Port=26
  m12 : Inport  Port=27
  m20 : Inport  Port=28
  m21 : Inport  Port=29
  m22 : Inport  Port=30
  Pt0 : Inport  Port=31
  Middle_Process : Subsystem
  Subsystem : Subsystem
  Subsystem1 : Subsystem
  RangeX : Outport
  VelX : Outport  Port=2
  RangeY : Outport  Port=3
  VelY : Outport  Port=4
  P11 : Outport  Port=5
  P12 : Outport  Port=6
  P13 : Outport  Port=7
  P14 : Outport  Port=8
  P21 : Outport  Port=9
  P22 : Outport  Port=10
  P23 : Outport  Port=11
  P24 : Outport  Port=12
  P31 : Outport  Port=13
  P32 : Outport  Port=14
  P33 : Outport  Port=15
  P34 : Outport  Port=16
  P41 : Outport  Port=17
  P42 : Outport  Port=18
  P43 : Outport  Port=19
  P44 : Outport  Port=20
  wires:
  Pre_vx/1 -> Subsystem1/2(Pre_vx)
  pre_p14/1 -> Subsystem1/8(pre_p14)
  m21/1 -> Subsystem1/29(m21)
  pre_p31/1 -> Subsystem1/13(pre_p31)
  pre_p13/1 -> Subsystem1/7(pre_p13)
  Pre_x/1 -> Subsystem1/1(Pre_x)
  pre_p41/1 -> Subsystem1/17(pre_p41)
  mk/1 -> Subsystem1/21(mk)
  pre_p21/1 -> Subsystem1/9(pre_p21)
  pre_p24/1 -> Subsystem1/12(pre_p24)
  pre_p11/1 -> Subsystem1/5(pre_p11)
  pre_p42/1 -> Subsystem1/18(pre_p42)
  pre_p32/1 -> Subsystem1/14(pre_p32)
  Pre_y/1 -> Subsystem1/3(Pre_y)
  Pre_vy/1 -> Subsystem1/4(Pre_vy)
  m20/1 -> Subsystem1/28(m20)
  m11/1 -> Subsystem1/26(m11)
  m00/1 -> Subsystem1/22(m00)
  m12/1 -> Subsystem1/27(m12)
  pre_p33/1 -> Subsystem1/15(pre_p33)
  pre_p44/1 -> Subsystem1/20(pre_p44)
  m2/1 -> Subsystem1/24(m2)
  pre_p34/1 -> Subsystem1/16(pre_p34)
  m10/1 -> Subsystem1/25(m10)
  pre_p12/1 -> Subsystem1/6(pre_p12)
  m01/1 -> Subsystem1/23(m01)
  pre_p22/1 -> Subsystem1/10(pre_p22)
  pre_p23/1 -> Subsystem1/11(pre_p23)
  m22/1 -> Subsystem1/30(m22)
  pre_p43/1 -> Subsystem1/19(pre_p43)
  Subsystem/1(RangeX) -> RangeX/1
  Middle_Process/1(Data) -> Subsystem/1(DataIn)
  Subsystem/2(VelX) -> VelX/1
  Subsystem/6(P12) -> P12/1
  Subsystem/4(VelY) -> VelY/1
  Subsystem/3(RangeY) -> RangeY/1
  Subsystem/5(P11) -> P11/1
  Subsystem1/1(Source) -> Middle_Process/1(Source)  "Source"
  Pt0/1 -> Subsystem1/31(Pt0)
  Subsystem/20(P44) -> P44/1
  Subsystem/13(P31) -> P31/1
  Subsystem/11(P23) -> P23/1
  Subsystem/14(P32) -> P32/1
  Subsystem/16(P34) -> P34/1
  Subsystem/18(P42) -> P42/1
  Subsystem/17(P41) -> P41/1
  Subsystem/19(P43) -> P43/1
  Subsystem/15(P33) -> P33/1
  Subsystem/10(P22) -> P22/1
  Subsystem/8(P14) -> P14/1
  Subsystem/12(P24) -> P24/1
  Subsystem/7(P13) -> P13/1
  Subsystem/9(P21) -> P21/1

== system ADU_Integration_Y2016_simulation/Fusion_Model/Fusion_Block/Global_Fusion/Fusion_Center/FusTrackPredict.Forecast/Predict/F ==
  DataIn : Inport
  Add : Sum  Inputs=++++
  F_line_1 : Subsystem
  F_line_2 : Subsystem
  F_line_3 : Subsystem
  F_line_4 : Subsystem
  F : Outport
  wires:
  DataIn/1 -> F_line_3/1(Data_in), F_line_1/1(Data_in)
  F_line_1/1(F_line_1) -> Add/1
  F_line_2/1(F_line_2) -> Add/2
  F_line_3/1(F_line_3) -> Add/3
  F_line_4/1(F_line_4) -> Add/4
  Add/1 -> F/1

== system ADU_Integration_Y2016_simulation/Fusion_Model/Fusion_Block/Global_Fusion/Fusion_Center/FusTrackPredict.Forecast/Predict/State_PreTime ==
  Source : Inport
  Bus Selector : BusSelector  OutputSignals=Pre_x,Pre_vx,Pre_y,Pre_vy
  Mux : Mux
  X_k : Outport
  wires:
  Source/1 -> Bus Selector/1
  Mux/1 -> X_k/1
  Bus Selector/1 -> Mux/1  "<Pre_x>"
  Bus Selector/3 -> Mux/3  "<Pre_y>"
  Bus Selector/4 -> Mux/4  "<Pre_vy>"
  Bus Selector/2 -> Mux/2  "<Pre_vx>"

== system ADU_Integration_Y2016_simulation/Fusion_Model/Fusion_Block/Global_Fusion/Fusion_Center/FusTrackUpdate.Update/Predict/Measurement ==
  Source : Inport
  Bus Selector : BusSelector  OutputSignals=Position_X[m],Position_Y[m]
  Mux : Mux  Inputs=2
  Z_k : Outport
  wires:
  Mux/1 -> Z_k/1
  Source/1 -> Bus Selector/1
  Bus Selector/1 -> Mux/1  "<Position_X[m]>"
  Bus Selector/2 -> Mux/2  "<Position_Y[m]>"

== system ADU_Integration_Y2016_simulation/Fusion_Model/Fusion_Block/Global_Fusion/Fusion_Center/FusTrackUpdate.Update/Predict/State_PreTime ==
  Source : Inport
  Bus Selector : BusSelector  OutputSignals=Pre_x,Pre_vx,Pre_y,Pre_vy
  Mux : Mux
  X_k : Outport
  wires:
  Source/1 -> Bus Selector/1
  Mux/1 -> X_k/1
  Bus Selector/2 -> Mux/2  "<Pre_vx>"
  Bus Selector/1 -> Mux/1  "<Pre_x>"
  Bus Selector/4 -> Mux/4  "<Pre_vy>"
  Bus Selector/3 -> Mux/3  "<Pre_y>"

== system ADU_Integration_Y2016_simulation/Fusion_Model/Fusion_Block/Side_Fusion/Side_Fusion/FusTrackPredict.Forecast/Predict/F ==
  DataIn : Inport
  Add : Sum  Inputs=++++
  F_line_1 : Subsystem
  F_line_2 : Subsystem
  F_line_3 : Subsystem
  F_line_4 : Subsystem
  F : Outport
  wires:
  DataIn/1 -> F_line_3/1(Data_in), F_line_1/1(Data_in)
  F_line_1/1(F_line_1) -> Add/1
  F_line_2/1(F_line_2) -> Add/2
  F_line_3/1(F_line_3) -> Add/3
  F_line_4/1(F_line_4) -> Add/4
  Add/1 -> F/1

== system ADU_Integration_Y2016_simulation/Fusion_Model/Fusion_Block/Side_Fusion/Side_Fusion/FusTrackPredict.Forecast/Predict/State_PreTime ==
  Source : Inport
  Bus Selector : BusSelector  OutputSignals=Pre_x,Pre_vx,Pre_y,Pre_vy
  Mux : Mux
  X_k : Outport
  wires:
  Source/1 -> Bus Selector/1
  Mux/1 -> X_k/1
  Bus Selector/1 -> Mux/1  "<Pre_x>"
  Bus Selector/3 -> Mux/3  "<Pre_y>"
  Bus Selector/4 -> Mux/4  "<Pre_vy>"
  Bus Selector/2 -> Mux/2  "<Pre_vx>"

== system ADU_Integration_Y2016_simulation/Fusion_Model/Fusion_Block/Side_Fusion/Side_Fusion/G_cal/Cal_1/Subsystem1 ==
  Stj : Inport
  Bus Creator : BusCreator  Inputs=4
  Constant : Constant  Value=[1;0]
  Constant1 : Constant  Value=[0;1]
  Demux1 : Demux  Outputs=2
  Demux2 : Demux  Outputs=2
  Product1 : Product  Multiplication=Matrix(*)  RndMeth=Zero
  Product2 : Product  Multiplication=Matrix(*)  RndMeth=Zero
  Stj_signal : Outport
  wires:
  Constant1/1 -> Product2/2
  Product2/1 -> Demux2/1
  Product1/1 -> Demux1/1
  Stj/1 -> Product2/1, Product1/1
  Constant/1 -> Product1/2
  Bus Creator/1 -> Stj_signal/1
  Demux1/2 -> Bus Creator/2  "21"
  Demux1/1 -> Bus Creator/1  "11"
  Demux2/1 -> Bus Creator/3  "12"
  Demux2/2 -> Bus Creator/4  "22"

== system ADU_Integration_Y2016_simulation/Fusion_Model/Fusion_Block/Side_Fusion/Side_Fusion/Tracker_Initial.VelocityMethod/Dmt/X_vector_Gen ==
  x_t : Inport
  x_m : Inport  Port=2
  vx_max : Inport  Port=3
  vx_min : Inport  Port=4
  ts : Inport  Port=5
  Compare To Constant : simulink/Logic and Bit Operations/Compare To Constant  relop=>=  const=0  OutDataTypeStr=uint8
  Compare To Constant1 : simulink/Logic and Bit Operations/Compare To Constant  relop=>=  const=0  OutDataTypeStr=uint8
  Constant1 : Constant  Value=0
  Constant2 : Constant  Value=0
  Divide : Product  Inputs=**
  Divide2 : Product  Inputs=**
  Multiport Switch : MultiPortSwitch  DataPortOrder=Zero-based contiguous  Inputs=2  zeroidx=on
  Multiport Switch1 : MultiPortSwitch  DataPortOrder=Zero-based contiguous  Inputs=2  zeroidx=on
  Subtract1 : Sum  Inputs=+-
  Subtract2 : Sum  Inputs=+-
  Subtract3 : Sum  Inputs=+-
  Subtract4 : Sum
  Subtract5 : Sum
  x_vector : Outport
  wires:
  x_t/1 -> Subtract3/1, Subtract2/2
  x_m/1 -> Subtract3/2, Subtract2/1
  vx_max/1 -> Divide/1
  ts/1 -> Divide2/1, Divide/2
  Subtract1/1 -> Multiport Switch/3, Compare To Constant/1
  Compare To Constant/1 -> Multiport Switch/1
  Subtract2/1 -> Subtract1/1
  Divide/1 -> Subtract1/2
  Subtract5/1 -> x_vector/1
  Constant1/1 -> Multiport Switch/2
  Multiport Switch/1 -> Subtract5/1
  Subtract3/1 -> Subtract4/1
  vx_min/1 -> Divide2/2
  Divide2/1 -> Subtract4/2
  Compare To Constant1/1 -> Multiport Switch1/1
  Multiport Switch1/1 -> Subtract5/2
  Subtract4/1 -> Multiport Switch1/3, Compare To Constant1/1
  Constant2/1 -> Multiport Switch1/2

== system ADU_Integration_Y2016_simulation/Fusion_Model/Fusion_Block/Side_Fusion/Side_Fusion/Tracker_Initial.VelocityMethod/Dmt/Y_vector_Gen1 ==
  y_t : Inport
  y_m : Inport  Port=2
  vy_max : Inport  Port=3
  vy_min : Inport  Port=4
  ts : Inport  Port=5
  Compare To Constant : simulink/Logic and Bit Operations/Compare To Constant  relop=>=  const=0  OutDataTypeStr=uint8
  Compare To Constant1 : simulink/Logic and Bit Operations/Compare To Constant  relop=>=  const=0  OutDataTypeStr=uint8
  Constant1 : Constant  Value=0
  Constant2 : Constant  Value=0
  Divide : Product  Inputs=**
  Divide2 : Product  Inputs=**
  Multiport Switch : MultiPortSwitch  DataPortOrder=Zero-based contiguous  Inputs=2  zeroidx=on
  Multiport Switch1 : MultiPortSwitch  DataPortOrder=Zero-based contiguous  Inputs=2  zeroidx=on
  Subtract1 : Sum  Inputs=+-
  Subtract2 : Sum  Inputs=+-
  Subtract3 : Sum  Inputs=+-
  Subtract4 : Sum
  Subtract5 : Sum
  y_vector : Outport
  wires:
  Constant2/1 -> Multiport Switch1/2
  Subtract4/1 -> Compare To Constant1/1, Multiport Switch1/3
  Multiport Switch1/1 -> Subtract5/2
  Compare To Constant1/1 -> Multiport Switch1/1
  Divide2/1 -> Subtract4/2
  vy_min/1 -> Divide2/2
  Subtract3/1 -> Subtract4/1
  Multiport Switch/1 -> Subtract5/1
  Constant1/1 -> Multiport Switch/2
  Subtract5/1 -> y_vector/1
  Divide/1 -> Subtract1/2
  Subtract2/1 -> Subtract1/1
  Compare To Constant/1 -> Multiport Switch/1
  Subtract1/1 -> Compare To Constant/1, Multiport Switch/3
  ts/1 -> Divide/2, Divide2/1
  vy_max/1 -> Divide/1
  y_m/1 -> Subtract2/1, Subtract3/2
  y_t/1 -> Subtract2/2, Subtract3/1

== system ADU_Integration_Y2016_simulation/Fusion_Model/Fusion_Block/Side_Fusion/Side_Fusion/Tracker_Initial.cos_cal/Reltive_Deg_Cal/Side_Length_Cal ==
  In1 : Inport
  Bus Creator2 : BusCreator  Inputs=3
  a_cal : Subsystem
  b_cal : Subsystem
  c_cal : Subsystem
  Out1 : Outport
  wires:
  c_cal/1(c) -> Bus Creator2/3  "c"
  Bus Creator2/1 -> Out1/1
  In1/1 -> c_cal/1(In1), b_cal/1(In1), a_cal/1(In1)
  a_cal/1(a) -> Bus Creator2/1  "a"
  b_cal/1(b) -> Bus Creator2/2  "b"

== system ADU_Integration_Y2016_simulation/Fusion_Model/Fusion_Block/Side_Fusion/Side_Fusion/Tracker_Update.Tracker_Filter.Update.Update/Model_Update/Middle_Process ==
  Source : Inport
  Bus Creator4 : BusCreator  Inputs=5
  Kalman_Gain : Subsystem
  S_Cal : Subsystem
  Subsystem : Subsystem
  Data : Outport
  wires:
  S_Cal/1(S) -> Bus Creator4/1, Kalman_Gain/1(S)
  Kalman_Gain/1(K) -> Bus Creator4/2
  Bus Creator4/1 -> Data/1
  Source/1 -> Subsystem/1(Source), Bus Creator4/3, Kalman_Gain/2(Source), S_Cal/1(Source)
  Subsystem/1(MeasureData) -> Bus Creator4/4  "MeasureGen"
  Subsystem/2(V) -> Bus Creator4/5
